simulink model "be2bis"  (R2013a)
settings: Solver=ode45  StartTime=0.0  StopTime=10.0  RelTol=1e-3
values from neighbouring files (symbols this model uses):
  f0 = 4.2*10^(-4)    (= 0.00042)    [variablesCC.m]
  f1 = 1.5 * 10^(-4)    (= 0.00015)    [variablesCC.m]
  g22 = 1/([0, -C]*([-R/L, -Kfem/L; Km/J, -f0/J]-[2*Valim/L;0]*Kt2)^(-1)*[2*Valim/L;0])    [variablesCC.m]
  J = 9.2 * 10^(-5)    (= 9.2e-05)    [variablesCC.m]
  Kfem = 60 * 10^(-3)    (= 0.06)    [variablesCC.m]
  Km = 60 * 10^(-3)    (= 0.06)    [variablesCC.m]
  Kr2 = K2emepart(3)    [variablesCC.m]
  Kt2 = K2emepart(1:2)    [variablesCC.m]
  L = 2.3 * 10 ^(-3)    (= 0.0023)    [variablesCC.m]
  R = 1.2    [variablesCC.m]
  Td = 250 * 10^(-6)    (= 0.00025)    [variablesCC.m]
  Valim = 35    [variablesCC.m]
libraries: simulink x1
settings Model: Creator=tfumey  LastModifiedBy=tfumey

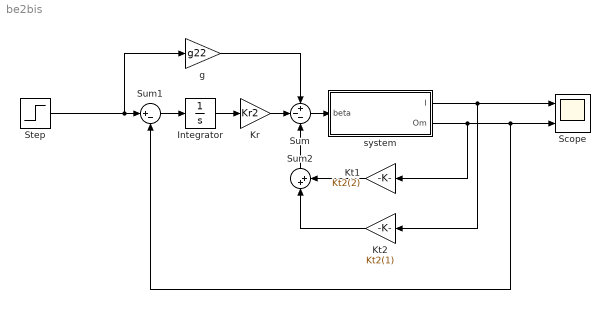
== system be2bis ==
  Integrator : Integrator
  Kr : Gain  Gain=Kr2
  "Kt1 " : Gain  Gain=Kt2(2)
  Kt2 : Gain  Gain=Kt2(1)
  Scope : Scope  NumInputPorts=2
      settings: YMin=-5~-5  YMax=5~5
  Step : Step  SampleTime=0
  Sum : Sum  Inputs=+--
  Sum1 : Sum  Inputs=|+-
  Sum2 : Sum  Inputs=|++
  g : Gain  Gain=g22
  system : Subsystem
  wires:
  Kr/1 -> Sum/2
  Sum/1 -> system/1(beta)
  Step/1 -> g/1, Sum1/1
  system/1(I) -> Kt2/1, Scope/1
  Integrator/1 -> Kr/1
  Sum1/1 -> Integrator/1
  g/1 -> Sum/1
  system/2(Om) -> "Kt1 "/1, Sum1/2, Scope/2
  Sum2/1 -> Sum/3
  "Kt1 "/1 -> Sum2/2
  Kt2/1 -> Sum2/1

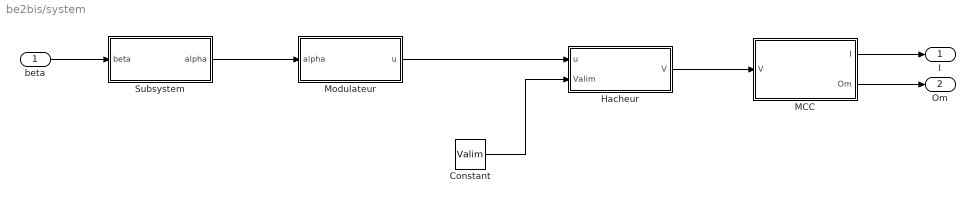
== system be2bis/system ==
  beta : Inport
  Constant : Constant  Value=Valim
  Hacheur : Subsystem
  MCC : Subsystem
  Modulateur : Subsystem
  Subsystem : Subsystem
  I : Outport
  Om : Outport  Port=2
  wires:
  beta/1 -> Subsystem/1(beta)
  Hacheur/1(V) -> MCC/1(V)
  Constant/1 -> Hacheur/2(Valim)
  Modulateur/1(u) -> Hacheur/1(u)
  MCC/1(I) -> I/1
  MCC/2(Om) -> Om/1
  Subsystem/1(alpha) -> Modulateur/1("alpha ")

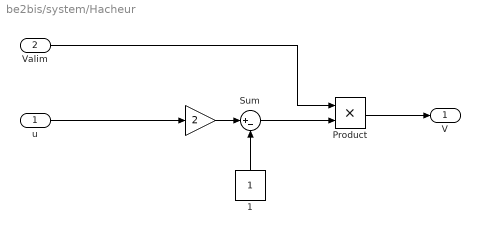
== system be2bis/system/Hacheur ==
  u : Inport
  Valim : Inport  Port=2
  " " : Gain  Gain=2
  1 : Constant
  Product : Product
  Sum : Sum  Inputs=|+-
  V : Outport
  wires:
  u/1 -> " "/1
  " "/1 -> Sum/1
  1/1 -> Sum/2
  Sum/1 -> Product/2
  Valim/1 -> Product/1
  Product/1 -> V/1

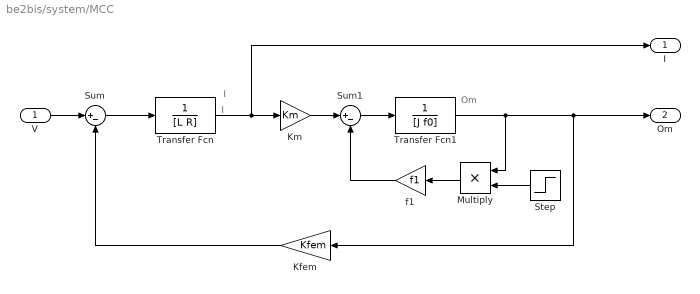
== system be2bis/system/MCC ==
  note: I
  note: I
  note: Om
  V : Inport
  Kfem : Gain  Gain=Kfem
  Km : Gain  Gain=Km
  Multiply : Product  Inputs=**
  Step : Step  Time=0.1  SampleTime=0
  Sum : Sum  Inputs=|+-
  Sum1 : Sum  Inputs=|+-
  Transfer Fcn : TransferFcn  Denominator=[L R]
  Transfer Fcn1 : TransferFcn  Denominator=[J f0]
  f1 : Gain  Gain=f1
  I : Outport
  Om : Outport  Port=2
  wires:
  V/1 -> Sum/1
  Kfem/1 -> Sum/2
  Sum/1 -> Transfer Fcn/1
  Transfer Fcn/1 -> I/1, Km/1
  Transfer Fcn1/1 -> Multiply/1, Om/1, Kfem/1
  Sum1/1 -> Transfer Fcn1/1
  Km/1 -> Sum1/1
  f1/1 -> Sum1/2
  Multiply/1 -> f1/1
  Step/1 -> Multiply/2

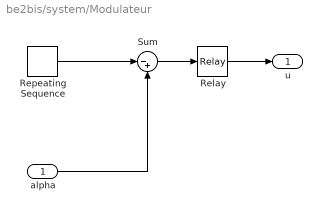
== system be2bis/system/Modulateur ==
  "alpha " : Inport
  Relay : Relay
  Repeating Sequence : simulink/Sources/Repeating Sequence  rep_seq_t=[0 Td]  rep_seq_y=[0 1]
  Sum : Sum  Inputs=|-+
  u : Outport
  wires:
  Repeating Sequence/1 -> Sum/1
  "alpha "/1 -> Sum/2
  Sum/1 -> Relay/1
  Relay/1 -> u/1

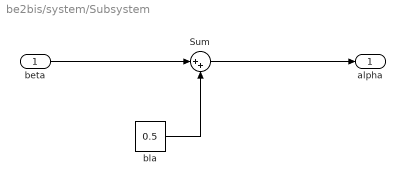
== system be2bis/system/Subsystem ==
  beta : Inport
  Sum : Sum  Inputs=|++
  bla : Constant  Value=0.5
  alpha : Outport
  wires:
  beta/1 -> Sum/1
  bla/1 -> Sum/2
  Sum/1 -> alpha/1
